simulink model "work_Unreal_demo2_VD"  (R2026a)
settings: Solver=ode23tb
model workspace (MAT data in the model file):
  SL_ROS_VariableLengthArrays_MaxSizes.CommonInfo.ArrayTruncateAction = 'EmitWarning'
  SL_ROS_VariableLengthArrays_MaxSizes.MsgTypeMap = containers.Map
  SL_ROS_VariableLengthArrays_MaxSizes.MsgTypeMap.serialization.keys = {'sensor_msgs/Image', 'sensor_msgs/PointCloud2'}
  SL_ROS_VariableLengthArrays_MaxSizes.MsgTypeMap.serialization.values{1}(1).PropertyName = 'data'
  SL_ROS_VariableLengthArrays_MaxSizes.MsgTypeMap.serialization.values{1}(1).DataType = 'uint8'
  SL_ROS_VariableLengthArrays_MaxSizes.MsgTypeMap.serialization.values{1}(1).MaxLength = 2764800
  SL_ROS_VariableLengthArrays_MaxSizes.MsgTypeMap.serialization.values{1}(2).PropertyName = 'encoding'
  SL_ROS_VariableLengthArrays_MaxSizes.MsgTypeMap.serialization.values{1}(2).DataType = 'uint8'
  SL_ROS_VariableLengthArrays_MaxSizes.MsgTypeMap.serialization.values{1}(2).MaxLength = 128
  SL_ROS_VariableLengthArrays_MaxSizes.MsgTypeMap.serialization.values{2}(1).PropertyName = 'data'
  SL_ROS_VariableLengthArrays_MaxSizes.MsgTypeMap.serialization.values{2}(1).DataType = 'uint8'
  SL_ROS_VariableLengthArrays_MaxSizes.MsgTypeMap.serialization.values{2}(1).MaxLength = 4915200
  SL_ROS_VariableLengthArrays_MaxSizes.MsgTypeMap.serialization.values{2}(2).PropertyName = 'fields'
  SL_ROS_VariableLengthArrays_MaxSizes.MsgTypeMap.serialization.values{2}(2).DataType = 'sensor_msgs/PointField'
  SL_ROS_VariableLengthArrays_MaxSizes.MsgTypeMap.serialization.values{2}(2).MaxLength = 16
  SL_ROS_VariableLengthArrays_MaxSizes.MsgTypeMap.serialization.uniformity = 0
  SL_ROS_VariableLengthArrays_MaxSizes.MsgTypeMap.serialization.keyType = 'char'
  SL_ROS_VariableLengthArrays_MaxSizes.MsgTypeMap.serialization.valueType = 'any'
undefined symbols (not defined in the file or in its folder): coder, ros, Sim3dSensor
libraries: autolibutils x4, ros2lib x4, vehdynlibtirecommon x3, sharedtransform x2, sim3dautolib x2, vehdynlibtire x1, sl_discontinuities x1, sim3dcameralib x1, sim3dphyssensorlib x1, sim3dlib x1
settings Model: Creator=akshran  LastModifiedBy=akshran
settings RTWCC: SystemTargetFile=ert.tlc  HardwareBoard=Robot Operating System 2 (ROS 2)  TLCOptions="-aInlineSetEventsForThisBaseRateFcn=TLC_FALSE -aSuppressMultiTaskScheduler=TLC_FALSE  -aRateBasedStepFcn=0"  Toolchain=Colcon Tools  TargetLang=C++  Description=Embedded Coder
settings ERTTargetCC: ExtModeTransport=2.0  ExtModeAutomaticAllocSize=off  RootIOFormat=Structure reference  CodeInterfacePackaging=C++ class

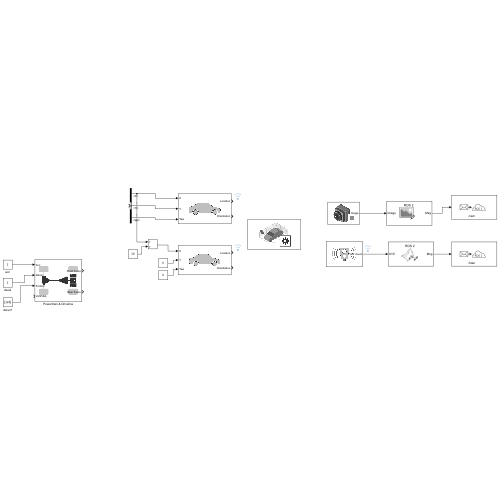
[thumbnail: Simulink's stored preview of the top-level diagram]
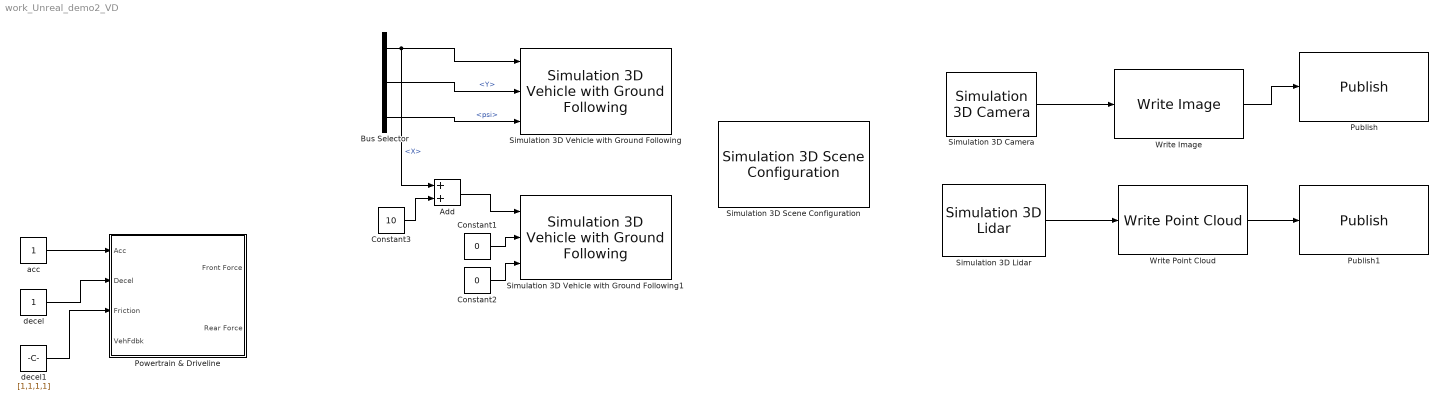
== system work_Unreal_demo2_VD ==
  Add : Sum
  Bus Selector : BusSelector  OutputSignals=InertFrm.Cg.Disp.X,InertFrm.Cg.Disp.Y,InertFrm.Cg.Ang.psi
  Constant1 : Constant  Value=0
  Constant2 : Constant  Value=0
  Constant3 : Constant  Value=10
  Powertrain & Driveline : Subsystem
      mask Display: image('vdbslibpt.png');
  Publish : ros2lib/Publish  topicSource=Specify your own  topic=/cam  messageType=sensor_msgs/Image  QOSHistory=Keep last  QOSDepth=10  QOSReliability=Reliable  QOSDurability=Volatile  QOSDeadline=Inf  QOSLifespan=Inf  QOSLiveliness=Automatic  QOSLeaseDuration=Inf  QOSAvoidROSNamespaceConventions=off
  Publish1 : ros2lib/Publish  topicSource=Specify your own  topic=/lidar  messageType=sensor_msgs/PointCloud2  QOSHistory=Keep last  QOSDepth=10  QOSReliability=Reliable  QOSDurability=Volatile  QOSDeadline=Inf  QOSLifespan=Inf  QOSLiveliness=Automatic  QOSLeaseDuration=Inf  QOSAvoidROSNamespaceConventions=off
  Simulation 3D Camera : sim3dcameralib/Simulation 3D Camera  Priority=1  sensorTag=Sim3dSensor�  sensorId=1  sensorName=Sim3dSensor�  vehTagList={'Custom ...';'Scene Origin';'SimulinkVehicle1';'SimulinkVehicle2'}  vehTag=SimulinkVehicle1  CoordinateSystem=ISO8855  mountLoc=Rearview mirror  offsetFlag=off  tmountOffset=[0, 0, 0]  extTmount=off  rmountOffset=[0, 0, 0]  extRmount=off  FocalLength=[1109, 1109]  OpticalCenter=[640, 360]  ImageSize=[720, 1280]  RadialDistortion=[0, 0]  TangentialDistortion=[0, 0]  SensorSkew=0  VisualizeFieldOfView=on  FieldOfViewRange=61  DepthOutportEnabled=off  SemanticOutportEnabled=off  TransformOutportEnabled=off  SampleTime=-1  mountPoint=[0.434 0 1.3]  mountOrientation=[0 0 0]  aMode=3  ID=1
      settings: LibrarySourceBlock=drivingsim3d/Simulation 3D Camera
  Simulation 3D Lidar : sim3dphyssensorlib/Simulation 3D Lidar  Priority=1  sensorTag=Sim3dSensor�  sensorId=2  sensorName=Sim3dSensor�  vehTagList={'Custom ...';'Scene Origin';'SimulinkVehicle1';'SimulinkVehicle2'}  vehTag=SimulinkVehicle1  CoordinateSystem=ISO8855  mountLoc=Roof center  offsetFlag=off  tmountOffset=[0, 0, 0]  rmountOffset=[0, 0, 0]  DetectionRange=120  RangeResolution=0.002  FieldOfViewSpecification=Symmetric  VerticalFOV=40  VerticalFOVBounds=single([-55 15])  VerticalResolution=1.25  VerticalSampleAngles=-20:20  HorizontalFOV=360  HorizontalFOVBounds=single([-180 180])  HorizontalResolution=0.16  HorizontalSampleAngles=-180:180  DistanceOutportEnabled=off  ReflectivityOutportEnabled=off  SemanticOutportEnabled=off  TransformOutportEnabled=off  SampleTime=-1  mountPoint=[-0.45 0 1.68]  mountOrientation=[0 0 0]  aMode=3  ID=2
      settings: LibrarySourceBlock=drivingsim3d/Simulation 3D Lidar
  Simulation 3D Scene Configuration : sim3dlib/Simulation 3D Scene Configuration  Priority=0  ProjectFormat=Default Scenes  SceneDesc=Straight road  ProjectName=C:\Program Files\MATLAB\R2026a\toolbox\shared\sim3d_projects\automotive_project_windows\UE\WindowsNoEditor\VehicleSimulation.exe  ScenePath=/Game/Maps/HwStrght  EnableOpenDRIVE=off  vehTagList={'Custom';'Scene Origin';'SimulinkVehicle1';'SimulinkVehicle2'}  vehTag=SimulinkVehicle1  AttachedCameraRelativeTranslation=[0 0 0]  FreeCameraDefaultInitialTranslation=[-6, 0, 2]  AttachedCameraRelativeRotation=[0, -15, 0]  FreeCameraDefaultInitialRotation=[0, -15, 0]  ViewpointName=Custom  FreeCameraInitialTranslation=[0, 0, 0]  FreeCameraInitialRotation=[0, 0, 0]  OpVisEn=off  Ts=1/60  EnableWindow=on  EnableRemoteAccess=off  SimulationMode=CoSimulation  SimulateUsing=Interpreted execution  EnableAnimationRecording=off  OverrideDefaultRecording=off  AnimationRecordingFileName=sim3dAnimation.mat  AnimationRecordingInterval=[0 inf]  EnableWeather=on  SunAzimuth=90  SunAltitude=40.0  EnableGeospatialSun=off  Latitude=0  Longitude=0  Date=2023-01-01  Time=10:30:00  GeoTimeZone=-5.0  SunDaylightSaving=off  wind=1  clouds=10  EnableVolumetricClouds=off  CloudCoverage=0  CloudAltitude=6  fog=20.0  rain=18.0  RaindropsEffect=off  SnowDensity=15.0  EnableGeospatial=off  TilesetSource=Earth terrain  UseTrueOrigin=off  OriginHeight=200  OriginLatitude=40.744652  OriginLongitude=-73.988864  MapStyle=Aerial  AdditionalAssetIDs=[]  UseAdvancedSunSky=off  SolarTime=11  TimeZone=-5  Day=21  Month=9  Year=2022  UseDaylightSavingTime=on  DSTStartDay=10  DSTStartMonth=3  DSTEndDay=3  DSTEndMonth=11  DSTSwitchHour=2  sensorTag=MainCamera1  sensorId=1  sensorName=MainCamera1  mountLoc=Origin  offsetFlag=off  tmountOffset=[0, 0, 0]  rmountOffset=[0, 0, 0]  HorizontalResolution=1280  VerticalResolution=720  HorizontalFOV=60  mountPoint=[0 0 0]  mountOrientation=[0 0 0]  aMode=3  ID=1  GeoTrigger=Inactive  ViewNameList={'Custom'}  ViewTranslationList={'[0 0 0]'}  ViewRotationList={'[0 0 0]'}
      settings: LibrarySourceBlock=drivingsim3d/Simulation 3D Scene Configuration
  Simulation 3D Vehicle with Ground Following : sim3dautolib/Simulation 3D Vehicle with Ground Following  Priority=-1  PassVehMesh=Sedan  MeshPath=/MathWorksAutomotiveContent/Vehicles/Muscle/Meshes/SK_MuscleCar.SK_MuscleCar  TrackWidth=1.9  WheelBase=3  WheelRadius=0.35  VehColor=Silver  CoordinateSystem=ISO8855  InitialPos=[0, 0, 0]  InitialRot=[0, 0, 0]  ActorName=SimulinkVehicle1  SampleTime=-1  ActorType=SimulinkVehicle  ID=1  aMode=3  ActorTag=SimulinkVehicle1  CoordinateScheme=0  VehLightsControl=off  HeadlightColor=[ 1, 1, 1 ]  HighBeamIntensity=100000  LowBeamIntensity=60000  HighBeamConeAngle=70  LowBeamConeAngle=70  LeftHeadlightOrientation=[ 0, 0 ]  RightHeadlightOrientation=[ 0, 0 ]  BrakelightIntensity=500  ReverselightIntensity=500  SignallightIntensity=500  SignallightPeriod=1  SignalPulseWidth=50  TransformOutportEnabled=on
      settings: LibrarySourceBlock=drivingsim3d/Simulation 3D Vehicle with Ground Following
  Simulation 3D Vehicle with Ground Following1 : sim3dautolib/Simulation 3D Vehicle with Ground Following  Priority=-1  PassVehMesh=Muscle car  MeshPath=/MathWorksAutomotiveContent/Vehicles/Muscle/Meshes/SK_MuscleCar.SK_MuscleCar  TrackWidth=1.9  WheelBase=3  WheelRadius=0.35  VehColor=Red  CoordinateSystem=ISO8855  InitialPos=[0, 0, 0]  InitialRot=[0, 0, 0]  ActorName=SimulinkVehicle2  SampleTime=-1  ActorType=SimulinkVehicle  ID=2  aMode=3  ActorTag=SimulinkVehicle2  CoordinateScheme=0  VehLightsControl=off  HeadlightColor=[ 1, 1, 1 ]  HighBeamIntensity=100000  LowBeamIntensity=60000  HighBeamConeAngle=70  LowBeamConeAngle=70  LeftHeadlightOrientation=[ 0, 0 ]  RightHeadlightOrientation=[ 0, 0 ]  BrakelightIntensity=500  ReverselightIntensity=500  SignallightIntensity=500  SignallightPeriod=1  SignalPulseWidth=50  TransformOutportEnabled=on
      settings: LibrarySourceBlock=drivingsim3d/Simulation 3D Vehicle with Ground Following
  Write Image : ros2lib/Write Image  ImageEncoding=rgb8  EncodingStruct=ros.msg.sensor_msgs.internal.ImageEncoding.info(coder.const('rgb8'))  HasAlpha=off  messageType=sensor_msgs/Image
  Write Point Cloud : ros2lib/Write Point Cloud  messageType=sensor_msgs/PointCloud2  Encoding=none  HasRGB=false  HasAlpha=false  HasIntensityCheck=off  HasIntensity=false  FieldNamesStruct=struct('x', 'single', 'y', 'single', 'z', 'single')
  acc : Constant
  decel : Constant
  decel1 : Constant  Value=[1,1,1,1]
  wires:
  Simulation 3D Camera/1 -> Write Image/1
  Simulation 3D Lidar/1 -> Write Point Cloud/1
  Write Image/1 -> Publish/1
  Write Point Cloud/1 -> Publish1/1
  Add/1 -> Simulation 3D Vehicle with Ground Following1/1
  Constant2/1 -> Simulation 3D Vehicle with Ground Following1/3
  Constant1/1 -> Simulation 3D Vehicle with Ground Following1/2
  Constant3/1 -> Add/2
  Bus Selector/1 -> Add/1, Simulation 3D Vehicle with Ground Following/1  "<X>"
  Bus Selector/2 -> Simulation 3D Vehicle with Ground Following/2  "<Y>"
  Bus Selector/3 -> Simulation 3D Vehicle with Ground Following/3  "<psi>"
  decel1/1 -> Powertrain & Driveline/3(Friction)
  acc/1 -> Powertrain & Driveline/1(Acc)
  decel/1 -> Powertrain & Driveline/2(Decel)

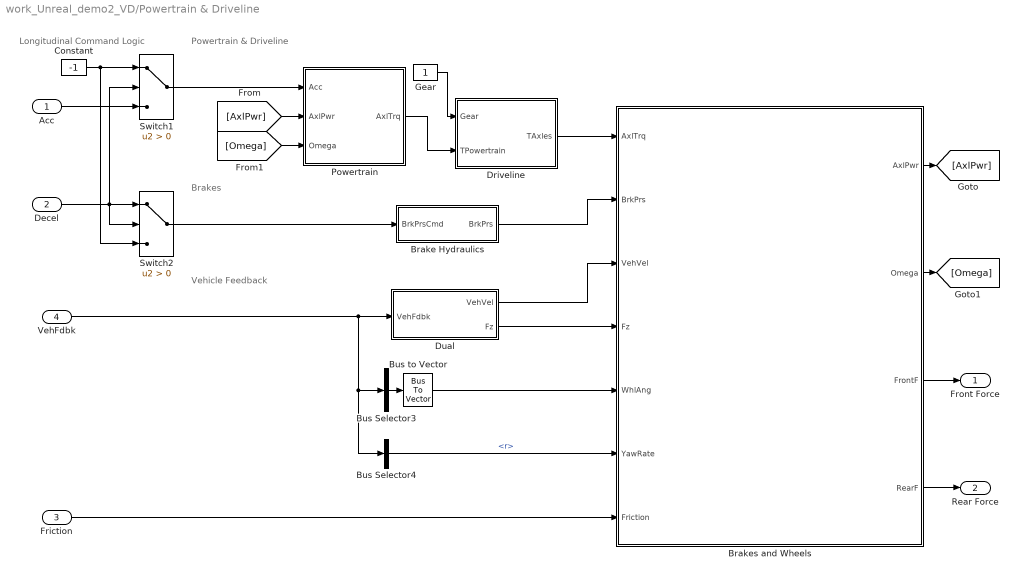
== system work_Unreal_demo2_VD/Powertrain & Driveline ==
  note: Longitudinal Command Logic
  note: Brakes
  note: Powertrain & Driveline
  note: Vehicle Feedback
  Acc : Inport
  Decel : Inport  Port=2
  Friction : Inport  Port=3
  VehFdbk : Inport  Port=4
  Brake Hydraulics : Subsystem
  Brakes and Wheels : Subsystem  TreatAsAtomicUnit=on
      mask Display: image('vdbslibwhls.png');
  Bus Selector3 : BusSelector  OutputSignals=BdyFrm.FrntAxl.Steer.WhlAngFL,BdyFrm.FrntAxl.Steer.WhlAngFR,BdyFrm.RearAxl.Steer.WhlAngRL,BdyFrm.RearAxl.Steer.WhlAngRR  OutputAsBus=on
  Bus Selector4 : BusSelector  OutputSignals=BdyFrm.Cg.AngVel.r
  Bus to Vector : BusToVector
  Constant : Constant  Value=-1
  Driveline : Subsystem  Variant=on  VariantControlMode=label  VariantControl=Variant1  LabelModeActiveChoice=0
  Dual : Subsystem  VariantControl=1
  Gear : Constant
  Powertrain : Subsystem
  Switch1 : Switch  Criteria=u2 > Threshold  SaturateOnIntegerOverflow=off  InputSameDT=off
  Switch2 : Switch  Criteria=u2 > Threshold  SaturateOnIntegerOverflow=off  InputSameDT=off
  Front Force : Outport  VectorParamsAs1DForOutWhenUnconnected=off
  Rear Force : Outport  Port=2  VectorParamsAs1DForOutWhenUnconnected=off
  wires:
  Decel/1 -> Switch1/2, Switch2/2, Switch2/1
  Acc/1 -> Switch1/3
  Constant/1 -> Switch2/3, Switch1/1
  Bus Selector3/1 -> Bus to Vector/1
  Switch1/1 -> Powertrain/1(Acc)
  Powertrain/1(AxlTrq) -> Driveline/2(TPowertrain)
  [AxlPwr] -> Powertrain/2(AxlPwr)
  [Omega] -> Powertrain/3(Omega)
  Switch2/1 -> Brake Hydraulics/1(BrkPrsCmd)
  Gear/1 -> Driveline/1(Gear)
  Friction/1 -> Brakes and Wheels/7(Friction)
  VehFdbk/1 -> Bus Selector4/1, Bus Selector3/1, Dual/1(VehFdbk)
  Brakes and Wheels/2(Omega) -> [Omega]
  Brakes and Wheels/3(FrontF) -> Front Force/1
  Brakes and Wheels/4(RearF) -> Rear Force/1
  Brakes and Wheels/1(AxlPwr) -> [AxlPwr]
  Bus to Vector/1 -> Brakes and Wheels/5(WhlAng)
  Dual/2(Fz) -> Brakes and Wheels/4(Fz)
  Bus Selector4/1 -> Brakes and Wheels/6(YawRate)  "<r>"
  Brake Hydraulics/1(BrkPrs) -> Brakes and Wheels/2(BrkPrs)
  Driveline/1(TAxles) -> Brakes and Wheels/1(AxlTrq)
  Dual/1(VehVel) -> Brakes and Wheels/3(VehVel)

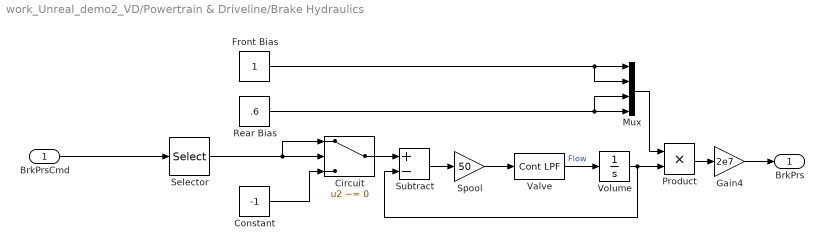
== system work_Unreal_demo2_VD/Powertrain & Driveline/Brake Hydraulics ==
  BrkPrsCmd : Inport
  Circuit : Switch  Criteria=u2 ~= 0  SaturateOnIntegerOverflow=off  InputSameDT=off
  Constant : Constant  Value=-1
  Front Bias : Constant
  Gain4 : Gain  Gain=2e7
  Mux : Mux
  Product : Product
  Rear Bias : Constant  Value=.6
  Selector : Selector  InputPortWidth=1  IndexOptions=Index vector (dialog)  Indices=[1 1 1 1]  OutputSizes=1
  Spool : Gain  Gain=50
  Subtract : Sum  Inputs=+-
  Valve : autolibutils/Cont LPF  wc=20*2*pi  AbsoluteTolerance=auto  aMode=2
  Volume : Integrator  LimitOutput=on  UpperSaturationLimit=1  LowerSaturationLimit=0
  BrkPrs : Outport  VectorParamsAs1DForOutWhenUnconnected=off
  wires:
  Volume/1 -> Subtract/2, Product/2
  Valve/1 -> Volume/1  "Flow"
  BrkPrsCmd/1 -> Selector/1
  Gain4/1 -> BrkPrs/1
  Circuit/1 -> Subtract/1
  Constant/1 -> Circuit/3
  Subtract/1 -> Spool/1
  Spool/1 -> Valve/1
  Front Bias/1 -> Mux/2, Mux/1
  Rear Bias/1 -> Mux/3, Mux/4
  Product/1 -> Gain4/1
  Mux/1 -> Product/1
  Selector/1 -> Circuit/1, Circuit/2

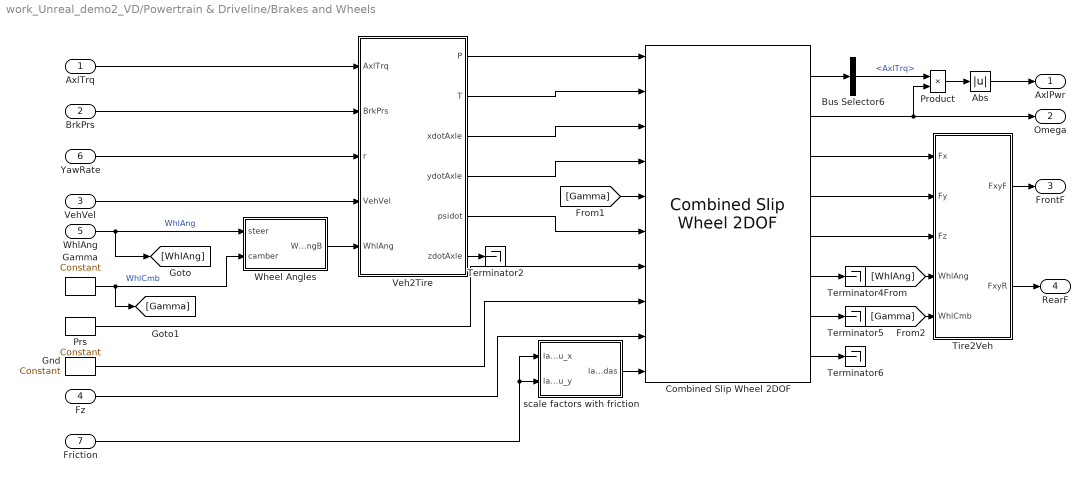
== system work_Unreal_demo2_VD/Powertrain & Driveline/Brakes and Wheels ==
  AxlTrq : Inport
  BrkPrs : Inport  Port=2
  VehVel : Inport  Port=3
  Fz : Inport  Port=4  PortDimensions=4
  WhlAng : Inport  Port=5
  YawRate : Inport  Port=6
  Friction : Inport  Port=7
  Abs : Abs  SaturateOnIntegerOverflow=off
  Bus Selector6 : BusSelector  OutputSignals=AxlTrq
  Combined Slip Wheel 2DOF : vehdynlibtire/Combined Slip Wheel 2DOF  tireType=Performance car 225/40R19  tireParamSet=vdynPassCar.mat  vertType=Magic Formula  plySteer=off  turnslip=off  BrakeType=Disc  mu_static=.3  mu_kinetic=.2  drum_abore=0.0508  drum_a=0.123  drum_c=0.212  drum_r=0.15  drum_theta1=0  drum_theta2=126  disk_abore=.05  Rm=.177  num_pads=2  brake_p_bpt=[1 11.4736842105263 21.9473684210526 32.4210526315789 42.8947368421053 53.3684210526316 63.8421052631579 74.3157894736842 84.7894736842105 95.2631578947368 105.736842105263 116.210526315789 126.684210526316 137.157894736842 147.631578947368 158.105263157895 168.578947368421 179.052631578947 189.526315789474 200]  brake_n_bpt=[0 52.6315789473684 105.263157894737 157.894736842105 210.526315789474 263.157894736842 315.789473684211 368.421052631579 421.052631578947 473.684210526316 526.315789473684 578.947368421053 631.578947368421 684.210526315789 736.842105263158 789.473684210526 842.105263157895 894.736842105263 947.368421052632 1000]  f_brake_t=[43.4900602404453 42.5056030554862 41.5350898940194 40.5780454442085 39.6340111501808 38.7025443887544 37.7832176914519 36.8756180088306 35.9793460143796 35.0940154454303 34.2192524787115 33.3546951383474 32.4999927342521 31.6548053290159 30.8188032315107 29.991666515561 29.1730845621415 28.362755623661 27.5603864089927 26.765691687993;498.991217495636 487.695866636631 476.560505099801 465.579679307235 454.748127933653 444.060772460445 433.51270824929 423.099196101319 412.81565427025 402.657650900201 392.620896861006 382.701238955775 372.894653477208 363.197240090814 353.605216024701 344.114910546964 334.722759712992 325.425301366216 316.219170376863 307.10109410434;954.492374750826 932.886130217776 911.585920305583 890.581313170261 869.862244717126 849.419000532136 829.242198807128 809.322774193808 789.651962526121 770.221286354971 751.0225412433 732.047782773203 713.289314220164 694.739674852612 676.391628817892 658.238154578366 640.272434863842 622.48784710877 604.877954344734 587.436496520688;1409.99353200602 1378.07639379892 1346.61133551136 1315.58294703329 1284.9763615006 1254.77722860383 1224.97168936497 1195.5463522863 1166.48827078199 1137.78492180974 1109.42418562559 1081.39432659063 1053.68397496312 1026.28210961441 999.178041611083 972.361398609768 945.822110014692 919.550392851325 893.536738312604 867.771898937035;1865.49468926121 1823.26665738007 1781.63675071715 1740.58458089631 1700.09047828407 1660.13545667552 1620.7011799228 1581.76993037878 1543.32457903786 1505.34855726451 1467.82583000789 1430.74087040806 1394.07863570608 1357.82454437621 1321.96445440427 1286.48464264117 1251.37178516554 1216.61293859388 1182.19552228048 1148.10730135338;2320.9958465164 2268.45692096121 2216.66216592293 2165.58621475934 2115.20459506754 2065.49368474721 2016.43067048064 1967.99350847127 1920.16088729373 1872.91219271928 1826.22747439018 1780.08741422549 1734.47329644903 1689.36697913801 1644.75086719747 1600.60788667257 1556.92146031639 1513.67548433643 1470.85430624835 1428.44270376973;2776.49700377159 2713.64718454235 2651.68758112871 2590.58784862237 2530.31871185102 2470.8519128189 2412.16016103848 2354.21708656376 2296.9971955496 2240.47582817405 2184.62911877248 2129.43395804292 2074.86795719199 2020.9094138998 1967.53727999066 1914.73113070398 1862.47113546724 1810.73803007899 1759.51309021622 1708.77810618608;3231.99816102678 3158.8374481235 3086.71299633449 3015.58948248539 2945.43282863449 2876.21014089059 2807.88965159632 2740.44066465625 2673.83350380547 2608.03946362882 2543.03076315477 2478.78050186034 2415.26261793494 2352.4518486616 2290.32369278385 2228.85437473538 2168.02081061809 2107.80057582154 2048.17187418409 1989.11350860242;3687.49931828197 3604.02771170464 3521.73841154027 3440.59111634842 3360.54694541796 3281.56836896228 3203.61914215416 3126.66424274874 3050.66981206134 2975.60309908359 2901.43240753707 2828.12704567777 2755.6572786779 2683.9942834234 2613.11010557704 2542.97761876678 2473.57048576894 2404.8631215641 2336.83065815196 2269.44891101877;4143.00047553716 4049.21797528579 3956.76382674606 3865.59275021144 3775.66106220143 3686.92659703397 3599.34863271199 3512.88782084123 3427.50612031721 3343.16673453836 3259.83405191936 3177.4735894952 3096.05193942085 3015.5367181852 2935.89651837023 2857.10086279818 2779.12016091979 2701.92566730665 2625.48944211983 2549.78431343512;4598.50163279235 4494.40823886693 4391.78924195184 4290.59438407447 4190.77517898491 4092.28482510566 3995.07812326983 3899.11139893372 3804.34242857308 3710.73036999313 3618.23569630166 3526.82013331263 3436.44660016381 3347.079152947 3258.68293116342 3171.22410682959 3084.66983607064 2998.98821304921 2914.1482260877 2830.11971585147;5054.00279004754 4939.59850244808 4826.81465715762 4715.59601793749 4605.88929576838 4497.64305317735 4390.80761382767 4285.3349770262 4181.17873682896 4078.2940054479 3976.63734068395 3876.16667713006 3776.84126090677 3678.62158770879 3581.46934395661 3485.34735086099 ...(+2764 chars)]  NOMPRES=262000  PRESMAX=1000000  PRESMIN=10000  FNOMIN=4600  FZMAX=9200  FZMIN=100  VXLOW=.01  KPUMAX=1.5  KPUMIN=-1.5  ALPMAX=1.5  ALPMIN=-1.5  CAMMAX=0.17453  CAMMIN=-0.17453  LONGVL=16.7  FxRelFreqLwrLim=200*pi  FyRelFreqLwrLim=200*pi  MyRelFreqLwrLim=100*pi  omegao=0  UNLOADED_RADIUS=0.33136  WIDTH=0.225  RIM_RADIUS=0.2413  ASPECT_RATIO=0.59239  MASS=10.35  IYY=0.99  br=1e-3  GRAVITY=-9.81  zo=0  zdoto=0  BREFF=8.25094594147963  DREFF=0.260468730454265  FREFF=0.0735298544471851  Q_RE0=1.00866439868088  Q_V1=0.000760413786224011  Q_V2=0.0463384792019201  Q_FZ1=0  Q_FZ2=15.6870832810226  Q_FZ3=0  Q_FCX=0.138643970247602  Q_FCY=0.10843499565426  Q_FCY2=-0.465763352339538  PFZ1=0.69958166705601  VERTICAL_STIFFNESS=207885.061134007  VERTICAL_DAMPING=494.649255786991  BOTTOM_OFFST=.01  BOTTOM_STIFF=2e6  Q_CAM1=0  Q_CAM2=0  Q_CAM3=0  Q_FYS1=0  Q_FYS2=0  Q_FYS3=0  LONGITUDINAL_STIFFNESS=388714.175879854  LATERAL_STIFFNESS=157087.404633332  PCFX1=0.18539229191199  PCFX2=0  PCFX3=0  PCFY1=0.163183345037677  PCFY2=0  PCFY3=0.249094918231954  Q_RA1=0.675942571700787  Q_RA2=0.73800463546164  Q_RB1=1.04487486456705  Q_RB2=-1.191763806629  PCX1=1.58523057950359  PDX1=1.0239116238178  PDX2=-0.0842405110022724  PDX3=0  PEX1=0.110312777158455  PEX2=0.313468516038146  PEX3=0  PEX4=0.0016060905760045  PKX1=21.3872544684023  PKX2=14.0006541873175  PKX3=-0.405326109653452  PHX1=0.000212599305364818  PHX2=0.00115950515263055  PVX1=1.59236164471432e-05  PVX2=0.000104321112127671  PPX1=-0.349461321276586  PPX2=0.387840040616429  PPX3=-0.0969947336569324  PPX4=0.0632271859795801  RBX1=12.7633329850276  RBX2=9.5787123658471  RBX3=0  RCX1=1.02796280922059  REX1=-0.45202516851367  REX2=-0.47304886171176  RHX1=0.000233272373115809  QSX1=-0.00788307788961443  QSX2=0.954629515459396  QSX3=0.0155855777667025  QSX4=0.125904607142414  QSX5=1.01110069703963  QSX6=20.1938577118433  QSX7=0.310818120717083  QSX8=-0.0430823751139655  QSX9=0.636494404888216  QSX10=0.142438060591663  QSX11=0.346766530036373  QSX12=0  QSX13=0  QSX14=0  PPMX1=0  PCY1=1.34299950037631  PDY1=0.878267729082195  PDY2=-0.0644597923147385  PDY3=0  PEY1=-0.809776534470972  PEY2=-0.600180598867198  PEY3=0.0991732552633487  PEY4=-6.5577974035573  PEY5=0  PKY1=-15.5714726518315  PKY2=1.73126522291751  PKY3=0.365349873517229  PKY4=1.98176755955416  PKY5=0  PKY6=-0.884005199550313  PKY7=-0.237259727611847  PHY1=-0.00183370557235628  PHY2=0.00346401302716671  PVY1=-0.00675427560163264  PVY2=0.036379218103843  PVY3=-0.163543984089166  PVY4=-0.491003349625726  PPY1=-0.62059646553185  PPY2=-0.0647824842338686  PPY3=-0.164648843290686  PPY4=0.283193909060098  PPY5=0  RBY1=10.7588809173639  RBY2=7.70420065295029  RBY3=3.40283755070691e-06  RBY4=0  RCY1=1.06691874059059  REY1=0.308244924574305  REY2=7.48775032604508e-06  RHY1=0.0118479204960415  RHY2=7.63650177161071e-06  RVY1=0.0560024425050078  RVY2=7.48487127056197e-06  RVY3=0  RVY4=98.4047026517149  RVY5=2.02759273900054  RVY6=15.7623064923347  QSY1=0.00699077564863536  QSY2=0  QSY3=0.00153535478298811  QSY4=8.55710322455322e-05  QSY5=0  QSY6=0  QSY7=0.89443879773793  QSY8=-0.403227641260894  QBZ1=11.666656027484  QBZ2=-1.30355438574485  QBZ3=0  QBZ4=0.177918305399071  QBZ5=-0.162481135068033  QBZ6=0  QBZ9=30.1445534682089  QBZ10=0  QCZ1=1.29026978207574  QDZ1=0.0886972644991399  QDZ2=-0.0058634820161856  QDZ3=0.3805597481383  QDZ4=0  QDZ6=0.00160914918118959  QDZ7=-0.00211036330862154  QDZ8=-0.13921904912557  QDZ9=0.00816585550028243  QDZ10=0  QDZ11=0  QEZ1=-2.19802254534746  QEZ2=1.01850535789165  QEZ3=0  QEZ4=0.278379679112054  QEZ5=-0.548414722765386  QHZ1=0.00148361198869669  QHZ2=0.00202017567585904  QHZ3=0.240316641332066  QHZ4=-0.210114035738085  PPZ1=-0.443927982388615  PPZ2=0  SSZ1=0.00914999585397887  SSZ2=0.0389830656052735  SSZ3=0  SSZ4=0  PDXP1=0.396718274678791  PDXP2=0  PDXP3=0  PKYP1=1.00587060633573  PDYP1=0.40483048923438  PDYP2=0  PDYP3=0  PDYP4=0  PHYP1=0.992731942067188  PHYP2=0.150352945499914  PHYP3=0  PHYP4=-3.98988682633674  PECP1=0.502379254513503  PECP2=0  QDTP1=10.0178654287947  QCRP1=0.200627747200702  QCRP2=0.0995735881599772  QBRP1=0.0997107127960717  QDRP1=1.01432910167423  QDRP2=0  aMode=2
  Gamma : vehdynlibtirecommon/Constant  const=0  numWheels=4
  Gnd : vehdynlibtirecommon/Constant  const=0  numWheels=4
  Product : Product
  Prs : vehdynlibtirecommon/Constant  const=2.4e5  numWheels=4
  Terminator{2,4..6} (4 alike) : Terminator
  Tire2Veh : Subsystem
  Veh2Tire : Subsystem
  Wheel Angles : Subsystem
  scale factors with friction : Subsystem  mask{numWheels=4}
      mask prompts: numWheels "Number of wheels"
  AxlPwr : Outport
  Omega : Outport  Port=2
  FrontF : Outport  Port=3
  RearF : Outport  Port=4
  wires:
  Gnd/1 -> Combined Slip Wheel 2DOF/8
  Combined Slip Wheel 2DOF/1 -> Bus Selector6/1
  Combined Slip Wheel 2DOF/2 -> Omega/1, Product/2
  Combined Slip Wheel 2DOF/7 -> Terminator5/1
  Combined Slip Wheel 2DOF/6 -> Terminator4/1
  Product/1 -> Abs/1
  Fz/1 -> Combined Slip Wheel 2DOF/9
  Veh2Tire/3(xdotAxle) -> Combined Slip Wheel 2DOF/3
  Combined Slip Wheel 2DOF/8 -> Terminator6/1
  Prs/1 -> Combined Slip Wheel 2DOF/7
  Friction/1 -> scale factors with friction/1(lamda_mu_x), scale factors with friction/2(lamda_mu_y)
  Abs/1 -> AxlPwr/1
  Bus Selector6/1 -> Product/1  "<AxlTrq>"
  scale factors with friction/1(lambdas) -> Combined Slip Wheel 2DOF/10
  Veh2Tire/5(psidot) -> Combined Slip Wheel 2DOF/6
  Combined Slip Wheel 2DOF/3 -> Tire2Veh/1(Fx)
  Combined Slip Wheel 2DOF/4 -> Tire2Veh/2(Fy)
  Combined Slip Wheel 2DOF/5 -> Tire2Veh/3(Fz)
  WhlAng/1 -> [WhlAng], Wheel Angles/1(steer)  "WhlAng"
  Gamma/1 -> [Gamma], Wheel Angles/2(camber)  "WhlCmb"
  Tire2Veh/1(FxyF) -> FrontF/1
  Tire2Veh/2(FxyR) -> RearF/1
  Veh2Tire/2(T) -> Combined Slip Wheel 2DOF/2
  BrkPrs/1 -> Veh2Tire/2(BrkPrs)
  AxlTrq/1 -> Veh2Tire/1(AxlTrq)
  Wheel Angles/1(WhlAngB) -> Veh2Tire/5(WhlAng)
  VehVel/1 -> Veh2Tire/4(VehVel)
  Veh2Tire/6(zdotAxle) -> Terminator2/1
  Veh2Tire/1(P) -> Combined Slip Wheel 2DOF/1
  Veh2Tire/4(ydotAxle) -> Combined Slip Wheel 2DOF/4
  YawRate/1 -> Veh2Tire/3(r)
  [WhlAng] -> Tire2Veh/4(WhlAng)
  [Gamma] -> Combined Slip Wheel 2DOF/5
  [Gamma] -> Tire2Veh/5(WhlCmb)

== system work_Unreal_demo2_VD/Powertrain & Driveline/Driveline ==
  Gear : Inport
  TPowertrain : Inport  Port=2  PortDimensions=1
  AWD : Subsystem  VariantControl=2
  FWD : Subsystem  VariantControl=1
  RWD : Subsystem  VariantControl=0
  TAxles : Outport  PortDimensions=4  VectorParamsAs1DForOutWhenUnconnected=off

== system work_Unreal_demo2_VD/Powertrain & Driveline/Dual ==
  VehFdbk : Inport
  Dual Fz : Subsystem
  Dual V : Subsystem
  VehVel : Outport  VectorParamsAs1DForOutWhenUnconnected=off
  Fz : Outport  Port=2  VectorParamsAs1DForOutWhenUnconnected=off
  wires:
  Dual V/1(Out1) -> VehVel/1
  VehFdbk/1 -> Dual Fz/1(In1), Dual V/1(In1)
  Dual Fz/1(Out1) -> Fz/1

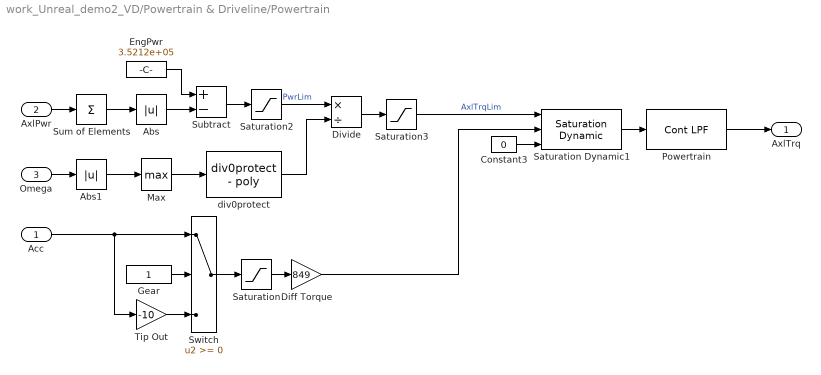
== system work_Unreal_demo2_VD/Powertrain & Driveline/Powertrain ==
  Acc : Inport
  AxlPwr : Inport  Port=2  PortDimensions=4
  Omega : Inport  Port=3  PortDimensions=4
  Abs : Abs  ZeroCross=off  SaturateOnIntegerOverflow=off
  Abs1 : Abs  ZeroCross=off  SaturateOnIntegerOverflow=off
  Constant3 : Constant  Value=0
  Diff Torque : Gain  Gain=849
  Divide : Product  Inputs=*/
  EngPwr : Constant  Value=3.5212e+05
  Gear : Constant  SampleTime=-1
  Max : MinMax  Function=max  ZeroCross=off
  Powertrain : autolibutils/Cont LPF  wc=3.5212e+05  AbsoluteTolerance=auto  aMode=2
  Saturation : Saturate  UpperLimit=inf  LowerLimit=0  ZeroCross=off
  Saturation Dynamic1 : sl_discontinuities/Saturation Dynamic  OutMin=[]  OutMax=[]  OutDataTypeStr=Inherit: Same as second input  OutDataType=fixdt(1, 16)  OutScaling=2^-10  DoSatur=off
  Saturation2 : Saturate  UpperLimit=inf  LowerLimit=100  ZeroCross=off
  Saturation3 : Saturate  UpperLimit=1000  LowerLimit=0  ZeroCross=off
  Subtract : Sum  Inputs=+-
  Sum of Elements : Sum  Inputs=+
  Switch : Switch  ZeroCross=off  SaturateOnIntegerOverflow=off  InputSameDT=off
  Tip Out : Gain  Gain=-10
  div0protect : autolibutils/div0protect - poly  thresh=1  ZeroCross1=on  aMode=2
  AxlTrq : Outport  VectorParamsAs1DForOutWhenUnconnected=off
  wires:
  Powertrain/1 -> AxlTrq/1
  Switch/1 -> Saturation/1
  Acc/1 -> Tip Out/1, Switch/1
  Saturation/1 -> Diff Torque/1
  Diff Torque/1 -> Saturation Dynamic1/2
  Gear/1 -> Switch/2
  Saturation Dynamic1/1 -> Powertrain/1
  Tip Out/1 -> Switch/3
  Constant3/1 -> Saturation Dynamic1/3
  Sum of Elements/1 -> Abs/1
  Abs/1 -> Subtract/2
  Divide/1 -> Saturation3/1
  div0protect/1 -> Divide/2
  Omega/1 -> Abs1/1
  Subtract/1 -> Saturation2/1
  Saturation2/1 -> Divide/1  "PwrLim"
  EngPwr/1 -> Subtract/1
  AxlPwr/1 -> Sum of Elements/1
  Saturation3/1 -> Saturation Dynamic1/1  "AxlTrqLim"
  Max/1 -> div0protect/1
  Abs1/1 -> Max/1

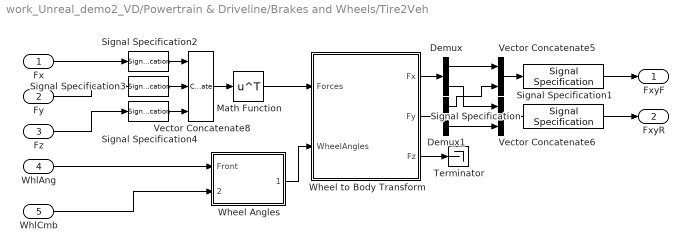
== system work_Unreal_demo2_VD/Powertrain & Driveline/Brakes and Wheels/Tire2Veh ==
  Fx : Inport
  Fy : Inport  Port=2
  Fz : Inport  Port=3
  WhlAng : Inport  Port=4
  WhlCmb : Inport  Port=5
  Demux : Demux  Outputs=[2,2]
  Demux1 : Demux  Outputs=[2,2]
  Math Function : Math  Operator=transpose  SignedPower=on
  Signal Specification : SignalSpecification  Unit=N
  Signal Specification1 : SignalSpecification  Unit=N
  Signal Specification2 : SignalSpecification  Dimensions=4
  Signal Specification3 : SignalSpecification  Dimensions=4
  Signal Specification4 : SignalSpecification  Dimensions=4
  Terminator : Terminator
  Vector Concatenate5 : Concatenate  Mode=Multidimensional array  ConcatenateDimension=2
  Vector Concatenate6 : Concatenate  Mode=Multidimensional array  ConcatenateDimension=2
  Vector Concatenate8 : Concatenate  NumInputs=3  Mode=Multidimensional array  ConcatenateDimension=2
  Wheel Angles : Subsystem
  Wheel to Body Transform : Subsystem
  FxyF : Outport
  FxyR : Outport  Port=2
  wires:
  Wheel Angles/1(Vehicle) -> Wheel to Body Transform/2(WheelAngles)
  Vector Concatenate5/1 -> Signal Specification1/1
  Demux/1 -> Vector Concatenate5/1
  Vector Concatenate8/1 -> Math Function/1
  Signal Specification1/1 -> FxyF/1
  Wheel to Body Transform/1(Fx) -> Demux/1
  Vector Concatenate6/1 -> Signal Specification/1
  Signal Specification4/1 -> Vector Concatenate8/3
  Demux1/2 -> Vector Concatenate6/2
  Wheel to Body Transform/2(Fy) -> Demux1/1
  Fy/1 -> Signal Specification3/1
  Math Function/1 -> Wheel to Body Transform/1(Forces)
  Wheel to Body Transform/3(Fz) -> Terminator/1
  Demux/2 -> Vector Concatenate6/1
  Signal Specification3/1 -> Vector Concatenate8/2
  Signal Specification2/1 -> Vector Concatenate8/1
  Demux1/1 -> Vector Concatenate5/2
  WhlAng/1 -> Wheel Angles/1(Front)
  Fx/1 -> Signal Specification2/1
  Fz/1 -> Signal Specification4/1
  Signal Specification/1 -> FxyR/1
  WhlCmb/1 -> Wheel Angles/2(Camber)

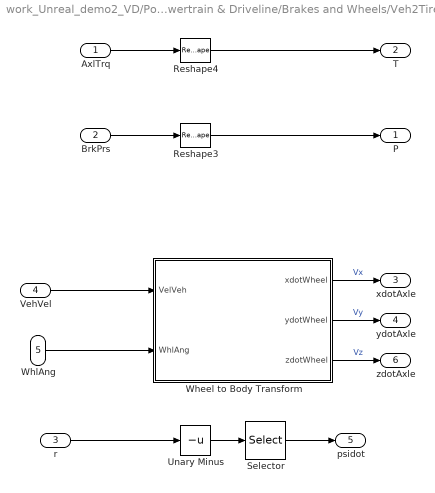
== system work_Unreal_demo2_VD/Powertrain & Driveline/Brakes and Wheels/Veh2Tire ==
  AxlTrq : Inport
  BrkPrs : Inport  Port=2
  r : Inport  Port=3
  VehVel : Inport  Port=4
  WhlAng : Inport  Port=5
  Reshape3 : Reshape
  Reshape4 : Reshape
  Selector : Selector  InputPortWidth=1  IndexOptions=Index vector (dialog)  Indices=[1 1 1 1]  OutputSizes=1
  Unary Minus : UnaryMinus
  Wheel to Body Transform : Subsystem
  P : Outport  VectorParamsAs1DForOutWhenUnconnected=off
  T : Outport  Port=2  VectorParamsAs1DForOutWhenUnconnected=off
  xdotAxle : Outport  Port=3  VectorParamsAs1DForOutWhenUnconnected=off
  ydotAxle : Outport  Port=4  VectorParamsAs1DForOutWhenUnconnected=off
  psidot : Outport  Port=5  VectorParamsAs1DForOutWhenUnconnected=off
  zdotAxle : Outport  Port=6  VectorParamsAs1DForOutWhenUnconnected=off
  wires:
  BrkPrs/1 -> Reshape3/1
  AxlTrq/1 -> Reshape4/1
  Wheel to Body Transform/1(xdotWheel) -> xdotAxle/1  "Vx"
  Wheel to Body Transform/2(ydotWheel) -> ydotAxle/1  "Vy"
  r/1 -> Unary Minus/1
  Reshape4/1 -> T/1
  VehVel/1 -> Wheel to Body Transform/1(VelVeh)
  Wheel to Body Transform/3(zdotWheel) -> zdotAxle/1  "Vz"
  Unary Minus/1 -> Selector/1
  Reshape3/1 -> P/1
  WhlAng/1 -> Wheel to Body Transform/2(WhlAng)
  Selector/1 -> psidot/1

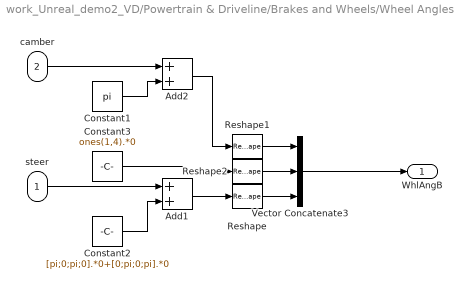
== system work_Unreal_demo2_VD/Powertrain & Driveline/Brakes and Wheels/Wheel Angles ==
  steer : Inport
  camber : Inport  Port=2
  Add1 : Sum
  Add2 : Sum
  Constant1 : Constant  Value=pi
  Constant2 : Constant  Value=[pi;0;pi;0].*0+[0;pi;0;pi].*0
  Constant3 : Constant  Value=ones(1,4).*0
  Reshape : Reshape  OutputDimensionality=Row vector (2-D)
  Reshape1 : Reshape  OutputDimensionality=Row vector (2-D)
  Reshape2 : Reshape  OutputDimensionality=Row vector (2-D)
  Vector Concatenate3 : Concatenate  NumInputs=3  Mode=Multidimensional array
  WhlAngB : Outport  VectorParamsAs1DForOutWhenUnconnected=off
  wires:
  Constant1/1 -> Add2/2
  Add2/1 -> Reshape1/1
  Add1/1 -> Reshape/1
  Reshape2/1 -> Vector Concatenate3/2
  Reshape1/1 -> Vector Concatenate3/1
  Constant3/1 -> Reshape2/1
  camber/1 -> Add2/1
  steer/1 -> Add1/1
  Reshape/1 -> Vector Concatenate3/3
  Vector Concatenate3/1 -> WhlAngB/1
  Constant2/1 -> Add1/2

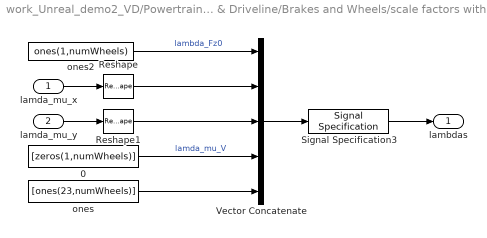
== system work_Unreal_demo2_VD/Powertrain & Driveline/Brakes and Wheels/scale factors with friction ==
  lamda_mu_x : Inport
  lamda_mu_y : Inport  Port=2
  0 : Constant  Value=[zeros(1,numWheels)]  VectorParams1D=off
  Reshape : Reshape  OutputDimensionality=Row vector (2-D)  OutputDimensions=[1,numWheels]
  Reshape1 : Reshape  OutputDimensionality=Row vector (2-D)  OutputDimensions=[1,numWheels]
  Signal Specification3 : SignalSpecification  Unit=1
  Vector Concatenate : Concatenate  NumInputs=5  Mode=Multidimensional array
  ones : Constant  Value=[ones(23,numWheels)]  VectorParams1D=off
  ones2 : Constant  Value=ones(1,numWheels)  VectorParams1D=off
  lambdas : Outport  Unit=1  VectorParamsAs1DForOutWhenUnconnected=off
  wires:
  lamda_mu_y/1 -> Reshape1/1
  lamda_mu_x/1 -> Reshape/1
  ones2/1 -> Vector Concatenate/1  "lambda_Fz0"
  Vector Concatenate/1 -> Signal Specification3/1
  ones/1 -> Vector Concatenate/5
  0/1 -> Vector Concatenate/4  "lamda_mu_V"
  Reshape1/1 -> Vector Concatenate/3
  Reshape/1 -> Vector Concatenate/2
  Signal Specification3/1 -> lambdas/1

== system work_Unreal_demo2_VD/Powertrain & Driveline/Driveline/AWD ==
  TPowertrain : Inport
  Gear : Inport  Port=2
  AWD : Gain  Gain=[1;1;1;1]./2
  Add : Sum
  Constant : Constant
  Constant1 : Constant  Value=zeros(4,1)
  Multiport Switch : MultiPortSwitch  DataPortOrder=Zero-based contiguous  zeroidx=on  SaturateOnIntegerOverflow=off  InputSameDT=off
  Unary Minus : UnaryMinus
  TAxles : Outport  VectorParamsAs1DForOutWhenUnconnected=off
  wires:
  TPowertrain/1 -> AWD/1
  Multiport Switch/1 -> TAxles/1
  Add/1 -> Multiport Switch/1
  Constant1/1 -> Multiport Switch/3
  AWD/1 -> Unary Minus/1, Multiport Switch/4
  Constant/1 -> Add/2
  Gear/1 -> Add/1
  Unary Minus/1 -> Multiport Switch/2

== system work_Unreal_demo2_VD/Powertrain & Driveline/Driveline/FWD ==
  TPowertrain : Inport
  Gear : Inport  Port=2
  Add : Sum
  Constant : Constant
  Constant1 : Constant  Value=zeros(4,1)
  FWD : Gain  Gain=[1;1;0;0]
  Multiport Switch : MultiPortSwitch  DataPortOrder=Zero-based contiguous  zeroidx=on  SaturateOnIntegerOverflow=off  InputSameDT=off
  Unary Minus : UnaryMinus
  TAxles : Outport  VectorParamsAs1DForOutWhenUnconnected=off
  wires:
  TPowertrain/1 -> FWD/1
  Multiport Switch/1 -> TAxles/1
  Add/1 -> Multiport Switch/1
  Constant1/1 -> Multiport Switch/3
  FWD/1 -> Unary Minus/1, Multiport Switch/4
  Constant/1 -> Add/2
  Gear/1 -> Add/1
  Unary Minus/1 -> Multiport Switch/2

== system work_Unreal_demo2_VD/Powertrain & Driveline/Driveline/RWD ==
  TPowertrain : Inport
  Gear : Inport  Port=2
  Add : Sum
  Constant : Constant
  Constant1 : Constant  Value=zeros(4,1)
  Multiport Switch : MultiPortSwitch  DataPortOrder=Zero-based contiguous  zeroidx=on  SaturateOnIntegerOverflow=off  InputSameDT=off
  RWD : Gain  Gain=[0;0;1;1]
  Unary Minus : UnaryMinus
  TAxles : Outport  VectorParamsAs1DForOutWhenUnconnected=off
  wires:
  RWD/1 -> Unary Minus/1, Multiport Switch/4
  TPowertrain/1 -> RWD/1
  Unary Minus/1 -> Multiport Switch/2
  Multiport Switch/1 -> TAxles/1
  Gear/1 -> Add/1
  Constant/1 -> Add/2
  Add/1 -> Multiport Switch/1
  Constant1/1 -> Multiport Switch/3

== system work_Unreal_demo2_VD/Powertrain & Driveline/Dual/Dual Fz ==
  In1 : Inport
  Add : Sum
  Bus Selector6 : BusSelector  OutputSignals=BdyFrm.Forces.Tires.FrntTires.Lft.Fz,BdyFrm.Forces.Tires.FrntTires.Rght.Fz,BdyFrm.Forces.Tires.RearTires.Lft.Fz,BdyFrm.Forces.Tires.RearTires.Rght.Fz
  Cont LPF : autolibutils/Cont LPF  wc=100*2*pi  AbsoluteTolerance=auto  aMode=2
  Saturation : Saturate  UpperLimit=10e3  LowerLimit=100  ZeroCross=off
  Unsprung Mass : Constant  Value=[0 0 80 80].*9.81
  Vector Concatenate : Concatenate  NumInputs=4
  Out1 : Outport  VectorParamsAs1DForOutWhenUnconnected=off
  wires:
  Saturation/1 -> Cont LPF/1
  Cont LPF/1 -> Add/1
  Vector Concatenate/1 -> Saturation/1
  Bus Selector6/2 -> Vector Concatenate/2  "<Fz>"
  Bus Selector6/1 -> Vector Concatenate/1  "<Fz>"
  Bus Selector6/3 -> Vector Concatenate/3  "<Fz>"
  Bus Selector6/4 -> Vector Concatenate/4  "<Fz>"
  Add/1 -> Out1/1
  Unsprung Mass/1 -> Add/2
  In1/1 -> Bus Selector6/1

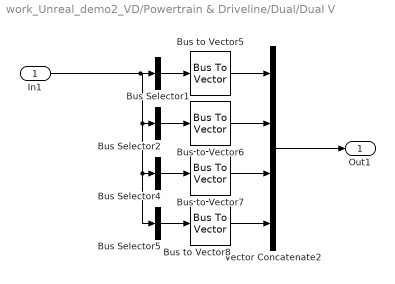
== system work_Unreal_demo2_VD/Powertrain & Driveline/Dual/Dual V ==
  In1 : Inport
  Bus Selector1 : BusSelector  OutputSignals=BdyFrm.FrntAxl.Lft.Vel.xdot,BdyFrm.FrntAxl.Lft.Vel.ydot,BdyFrm.FrntAxl.Lft.Vel.zdot  OutputAsBus=on
  Bus Selector2 : BusSelector  OutputSignals=BdyFrm.FrntAxl.Rght.Vel.xdot,BdyFrm.FrntAxl.Rght.Vel.ydot,BdyFrm.FrntAxl.Rght.Vel.zdot  OutputAsBus=on
  Bus Selector4 : BusSelector  OutputSignals=BdyFrm.RearAxl.Lft.Vel.xdot,BdyFrm.RearAxl.Lft.Vel.ydot,BdyFrm.RearAxl.Lft.Vel.zdot  OutputAsBus=on
  Bus Selector5 : BusSelector  OutputSignals=BdyFrm.RearAxl.Rght.Vel.xdot,BdyFrm.RearAxl.Rght.Vel.ydot,BdyFrm.RearAxl.Rght.Vel.zdot  OutputAsBus=on
  Bus to Vector{5..8} (4 alike) : BusToVector
  Vector Concatenate2 : Concatenate  NumInputs=4  Mode=Multidimensional array  ConcatenateDimension=2
  Out1 : Outport  VectorParamsAs1DForOutWhenUnconnected=off
  wires:
  Bus to Vector6/1 -> Vector Concatenate2/2
  Bus Selector2/1 -> Bus to Vector6/1
  Bus to Vector8/1 -> Vector Concatenate2/4
  Bus Selector4/1 -> Bus to Vector7/1
  Bus to Vector5/1 -> Vector Concatenate2/1
  Bus Selector1/1 -> Bus to Vector5/1
  In1/1 -> Bus Selector1/1, Bus Selector2/1, Bus Selector4/1, Bus Selector5/1
  Bus Selector5/1 -> Bus to Vector8/1
  Bus to Vector7/1 -> Vector Concatenate2/3
  Vector Concatenate2/1 -> Out1/1

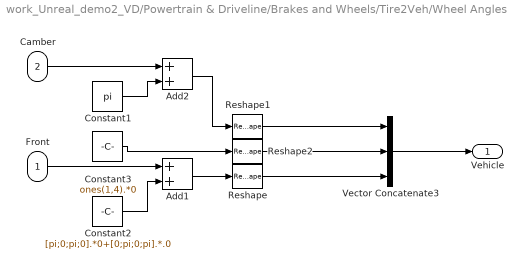
== system work_Unreal_demo2_VD/Powertrain & Driveline/Brakes and Wheels/Tire2Veh/Wheel Angles ==
  Front : Inport
  Camber : Inport  Port=2
  Add1 : Sum
  Add2 : Sum
  Constant1 : Constant  Value=pi
  Constant2 : Constant  Value=[pi;0;pi;0].*0+[0;pi;0;pi].*.0
  Constant3 : Constant  Value=ones(1,4).*0
  Reshape : Reshape  OutputDimensionality=Row vector (2-D)
  Reshape1 : Reshape  OutputDimensionality=Row vector (2-D)
  Reshape2 : Reshape  OutputDimensionality=Row vector (2-D)
  Vector Concatenate3 : Concatenate  NumInputs=3  Mode=Multidimensional array
  Vehicle : Outport  VectorParamsAs1DForOutWhenUnconnected=off
  wires:
  Constant1/1 -> Add2/2
  Reshape/1 -> Vector Concatenate3/3
  Reshape2/1 -> Vector Concatenate3/2
  Front/1 -> Add1/1
  Add2/1 -> Reshape1/1
  Add1/1 -> Reshape/1
  Constant3/1 -> Reshape2/1
  Reshape1/1 -> Vector Concatenate3/1
  Constant2/1 -> Add1/2
  Camber/1 -> Add2/1
  Vector Concatenate3/1 -> Vehicle/1

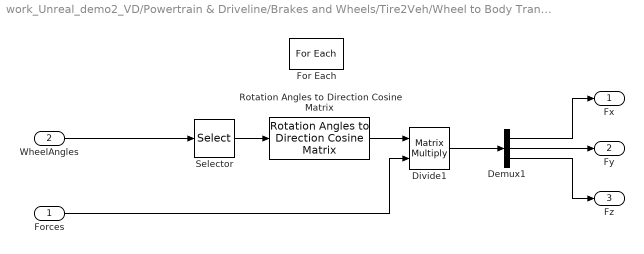
== system work_Unreal_demo2_VD/Powertrain & Driveline/Brakes and Wheels/Tire2Veh/Wheel to Body Transform ==
  Forces : Inport  PortDimensions=[3,1]  Partition=on  PartitionDimension=2  PartitionWidth=1  PartitionOffset=0
  WheelAngles : Inport  Port=2  Partition=on  PartitionDimension=2  PartitionWidth=1  PartitionOffset=0
  Demux1 : Demux  Outputs=3
  Divide1 : Product  Inputs=**  Multiplication=Matrix(*)
  For Each : ForEach  DisableCoverage=on
  Rotation Angles to Direction Cosine Matrix : sharedtransform/Rotation Angles to Direction Cosine Matrix  rotationOrder=ZYX  aMode=2
  Selector : Selector  InputPortWidth=3  IndexOptions=Index vector (dialog)  Indices=[3 2 1]  OutputSizes=1
  Fx : Outport  ConcatenationDimension=1  VectorParamsAs1DForOutWhenUnconnected=off
  Fy : Outport  Port=2  ConcatenationDimension=1  VectorParamsAs1DForOutWhenUnconnected=off
  Fz : Outport  Port=3  ConcatenationDimension=1  VectorParamsAs1DForOutWhenUnconnected=off
  wires:
  Divide1/1 -> Demux1/1
  Demux1/1 -> Fx/1
  Demux1/2 -> Fy/1
  Demux1/3 -> Fz/1
  Rotation Angles to Direction Cosine Matrix/1 -> Divide1/1
  Forces/1 -> Divide1/2
  WheelAngles/1 -> Selector/1
  Selector/1 -> Rotation Angles to Direction Cosine Matrix/1

== system work_Unreal_demo2_VD/Powertrain & Driveline/Brakes and Wheels/Veh2Tire/Wheel to Body Transform ==
  VelVeh : Inport  Partition=on  PartitionDimension=2  PartitionWidth=1  PartitionOffset=0
  WhlAng : Inport  Port=2  Partition=on  PartitionDimension=2  PartitionWidth=1  PartitionOffset=0
  Demux1 : Demux  Outputs=3
  Divide1 : Product  Inputs=**  Multiplication=Matrix(*)
  For Each : ForEach  DisableCoverage=on
  Rotation Angles to Direction Cosine Matrix : sharedtransform/Rotation Angles to Direction Cosine Matrix  rotationOrder=ZYX  aMode=2
  Selector : Selector  InputPortWidth=3  IndexOptions=Index vector (dialog)  Indices=[3 2 1]  OutputSizes=1
  xdotWheel : Outport  ConcatenationDimension=1  VectorParamsAs1DForOutWhenUnconnected=off
  ydotWheel : Outport  Port=2  ConcatenationDimension=1  VectorParamsAs1DForOutWhenUnconnected=off
  zdotWheel : Outport  Port=3  ConcatenationDimension=1  VectorParamsAs1DForOutWhenUnconnected=off
  wires:
  Divide1/1 -> Demux1/1
  Demux1/1 -> xdotWheel/1
  Demux1/2 -> ydotWheel/1
  Demux1/3 -> zdotWheel/1
  Rotation Angles to Direction Cosine Matrix/1 -> Divide1/1
  VelVeh/1 -> Divide1/2
  WhlAng/1 -> Selector/1
  Selector/1 -> Rotation Angles to Direction Cosine Matrix/1
